simulink model "full_simulation"  (R2025b)
settings: Solver=VariableStepAuto  StopTime=2000
values from neighbouring files (symbols this model uses):
  s = sensors.gyro.scaleFactor    [detumbling_Simulation_cuerpo_ABC.m]    (also in pucp_orbit_propagator.m = z / r_norm; test_PUCP_1.m = z / r_norm)
undefined symbols (not defined in the file or in its folder): Adaptive_controler, deg, dow, eu, I, IAU, InitialCondition, K, k_bdot, Ley_adaptacion, P, rad, reference_euler, w_r, w_s
libraries: aerolibconvert2 x6, matrix_library x4, sharedtransform x3, aerolibutil x2, simulink_extras x2, aerolibtransform2 x1
settings Model: Creator=b_ant  LastModifiedBy=b_ant
settings ConfigComp: PLC_TargetIDE=codesys35  PLC_MultiTBSigbuilderTimeRange=off  PLC_FoldFBCallOutputVar=off  PLC_RemoveUnusedSSMethodCallArguments=off  PLC_UseCallOutputArgSyntax=off  PLC_EnableUnsignedAndDoubleTypes=off  PLC_EnableUDTSplitting=off  PLC_MaxFieldsInUDT=500.0  PLC_InlineEnumCastFunction=off  PLC_RTWMaxIdLength=31.0  PLC_RollThreshold=5.0  PLC_ActiveTab=0.0  PLC_EnableStringLiteralTB=on  PLC_Enable64bitIntSupport=off
settings SimscapeCC: SimscapeNominalValues="[{\"value\":\"1\",\"unit\":\"A\"},{\"value\":\"1\",\"unit\":\"bar\"},{\"value\":\"1\",\"unit\":\"cm^2\"},{\"value\":\"1\",\"unit\":\"cm^3/s\"},{\"value\":\"1\",\"unit\":\"kJ/kg\"},{\"value\":\"1\",\"unit\":\"kW\"},{\"value\":\"1\",\"unit\":\"l\"},{\"value\":\"1\",\"unit\":\"N\"},{\"value\":\"1\",\"unit\":\"N*m\"},{\"value\":\"1\",\"unit\":\"V\"},{\"value\":\"0.001\",\"unit\":\"Wb\"}]"  SimscapeLogType=all  SimscapeLogDataHistory=10000.0

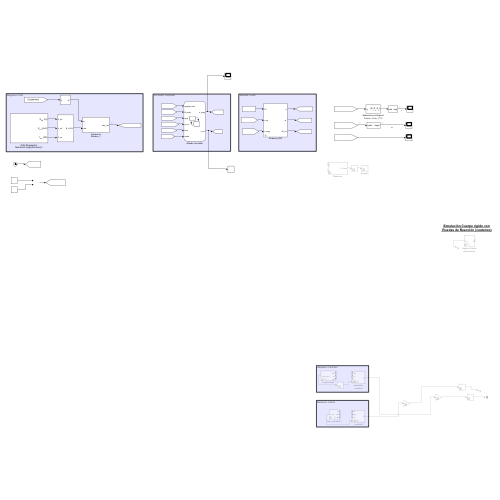
[thumbnail: Simulink's stored preview of the top-level diagram]
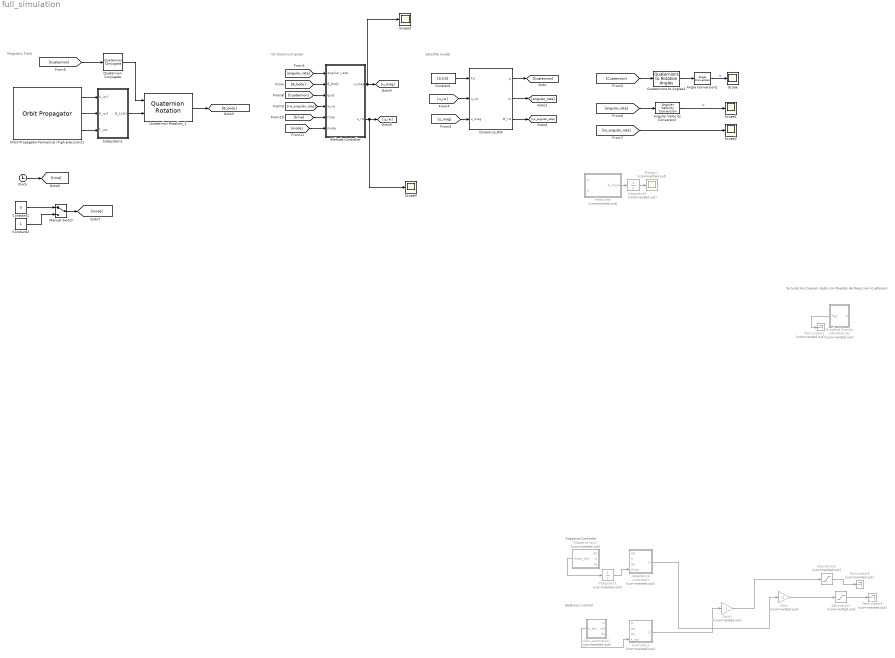
== system full_simulation ==
  note: Satellite model
  note: On board computer
  note: Magnetic Field
  note: Boskovic control
  note: Adaptive Controler
  note: Simulación Cuerpo rígido con
      | Ruedas de Reacción (cuatenos)
  Adaptative controler1 : Subsystem  Commented=on  mask{J=[1,1,1,0,0,0], lambda=1, kd=1}
      mask prompts: J "[Jcxx,Jcyy,Jczz,Jcxy,Jcxz,Jcyz]:"
      mask TypeOptions J: J/Value
      mask TypeOptions lambda: lambda/Value
      mask TypeOptions kd: Kd/Value
      mask DialogControl DescGroupVar Prompt: Adaptive controler
      mask DialogControl Control2 Prompt: Modeled inertia tensor:
      mask DialogControl H Prompt: Gains
  Adaptive law1 : Subsystem  Commented=on  mask{gamma=0.001, Lambda=1}
      mask TypeOptions gamma: gamma/Value
      mask TypeOptions Lambda: lambda/Value
  Angle Conversion2 : aerolibconvert2/Angle Conversion  IU=rad  OU=deg
  Angular Velocity Conversion : aerolibconvert2/Angular Velocity Conversion  IU=rad/s  OU=deg/s
  Attitude Controller : Stateflow chart  TreatAsAtomicUnit=on
  Clock : Clock
  Constant : Constant  Value=[0,0,0]
  Constant1 : Constant  Value=0
  Constant2 : Constant
  Controler1 : Subsystem  Commented=on  mask{delta=1, Umax=1.343*10^(-2)}
      mask TypeOptions delta: delta/Value
      mask TypeOptions Umax: Umax/Value
      mask DialogControl DescGroupVar Prompt: Boskovic Control
      mask DialogControl Control2 Prompt: Delta:
      mask DialogControl Control3 Prompt: Umax:
  Dinamica_RW : Subsystem  mask{I=I, Ang=eu, W=w_s, Wrw=w_r, dimensiones=dow}
      mask prompts: I "[Ix,Iy,Iz,Ixy,Ixz,Iyz] :"; Ang "[roll,pitch,yaw]:"; W "[Wx,Wy,Wz]"; Wrw "[Wrwx,Wrwy,Wrwz]"; dimensiones "[Ancho,Masa,Radio]:"
      mask TypeOptions I: I/Value
      mask TypeOptions Ang: Ang/Value
      mask TypeOptions W: W/Value
      mask TypeOptions Wrw: Wrw/Value
      mask TypeOptions dimensiones: dimentions/Value
      mask DialogControl Container3 Prompt: Tensor de Inercia
      mask DialogControl Container2 Prompt: Condiciones iniciales
      mask DialogControl Container4 Prompt: Ruedas de Reacción:
      mask DialogControl Control1 Prompt: Dimensiones:
  Energy1 : Scope  Commented=on
      settings: TimeSpan=10  ActiveDisplayYMinimum=0  ActiveDisplayYMaximum=2.75  DataLoggingVariableName=Energia3  DataLoggingSaveFormat=Array
  Gain : Gain  Commented=on  Gain=-1
  Gain1 : Gain  Commented=on  Gain=-1
  Gain_estimator1 : Subsystem  Commented=on  mask{delta=1, gamma=0.001, Umax=1.343*10^(-2), InitialCondition=1}
      mask prompts: InitialCondition "Simulink:blkprm_prompts:IntegratorInitCond"
      mask TypeOptions delta: delta/Value
      mask TypeOptions gamma: gamma/Value
      mask TypeOptions Umax: Umax/Value
      mask TypeOptions InitialCondition: Integrator/InitialCondition
      mask DialogControl DescGroupVar Prompt: Gain_estimator
      mask DialogControl Control2 Prompt: Gains:
      mask DialogControl Control3 Prompt: Initial Gain:
      mask DialogControl InitialCondition Prompt: Initial condition:
  Gradient Gravity disturbances : Subsystem  Commented=on  mask{J_tilde=[8.46,8.46,8.46,1.1,1.5,1.6]*10^(-3), rc=(6371+100)*10^(3), Drw=[0.015,0.025,0.043]}
      mask prompts: J_tilde "Satellite Inertia Tensor:"; rc "Distance from the center of the earth:"; Drw "Reaction wheels dimentions"
      mask TypeOptions J_tilde: J_tilde/Value
      mask TypeOptions rc: rc/Value
      mask TypeOptions Drw: dimentions/Value
      mask DialogControl DescGroupVar Prompt: Gravity gradient Torque
  Integrator1 : Integrator  Commented=on  InitialCondition=[1,1,1,0,0,0]
  Integrator3 : Integrator  Commented=on
  Manual Switch : ManualSwitch
  Measures : Subsystem  Commented=on
  Orbit Propagator Numerical (high precision)1 : OrbitPropagator  accelFrame=Fixed-frame  outportFrame=Fixed-frame  semiMajorAxis=orbit.semiMajorAxis  eccentricity=orbit.eccentricity  inclination=orbit.inclination  raan=orbit.rightAscensionOfAscendingNode  argPeriapsis=orbit.argumentOfPeriapsis  trueAnomaly=orbit.trueAnomaly  inertialPosition=[3649700.0 3308200.0 -4676600.0]  inertialVelocity=[-2750.8 6666.4 2573.4]  fixedPosition=[-4142689.0 -2676864.7 -4669861.6]  fixedVelocity=[1452.7 -6720.7 2568.1]  gravityModel=None  customR=3396200  customMu=4.305e13  customJ2=1.0826269e-03  customOmega=4.06125949e-3  outputTransform=on
  Quaternion Conjugate : aerolibutil/Quaternion Conjugate
  Quaternion Rotation_1 : aerolibutil/Quaternion Rotation
  Quaternions to Angles2 : sharedtransform/Quaternions to Rotation Angles  rotationOrder=ZYX  aMode=aMode
  Saturation1 : Saturate  Commented=on  UpperLimit=1.343*10^(-2)  LowerLimit=-1.343*10^(-2)
  Saturation2 : Saturate  Commented=on  UpperLimit=1.343*10^(-2)  LowerLimit=-1.343*10^(-2)
  Scope{,1..4} (5 alike) : Scope
      Scope settings: ActiveDisplayYMinimum=-23.210840938697004  ActiveDisplayYMaximum=43.99322143114955
      Scope1 settings: ActiveDisplayYMinimum=-0.62287287742311848  ActiveDisplayYMaximum=1.7831039675067617
      Scope2 settings: DataLoggingVariableName=ScopeData2
      Scope3 settings: ActiveDisplayYMinimum=-3.3528933558992531E-7  ActiveDisplayYMaximum=3.2851122357621673E-7  DataLoggingVariableName=ScopeData3
      Scope4 settings: ActiveDisplayYMinimum=-2.4173536825278268E-5  ActiveDisplayYMaximum=5.4003519984842569E-6  DataLoggingVariableName=ScopeData4
  Subsystem1 : Subsystem
  Terminator1 : Terminator  Commented=on
  Terminator4 : Terminator  Commented=on
  Terminator6 : Terminator  Commented=on
  wires:
  Quaternions to Angles2/1 -> Angle Conversion2/1
  Integrator3/1 -> Energy1/1
  Saturation2/1 -> Terminator6/1
  Integrator1/1 -> Adaptative controler1/4(theta)
  Controler1/1(U) -> Gain1/1
  Adaptive law1/1(theta_dot) -> Integrator1/1
  Gain/1 -> Saturation1/1
  Measures/1("K, theta") -> Integrator3/1
  Gain_estimator1/1(k_est) -> Controler1/4(K_est)
  Adaptative controler1/1(U) -> Gain/1
  Gain1/1 -> Saturation2/1
  Saturation1/1 -> Terminator4/1
  Angle Conversion2/1 -> Scope/1  "q"
  Gradient Gravity disturbances/1(Tgg) -> Terminator1/1
  Orbit Propagator Numerical (high precision)1/1 -> Subsystem1/1(X_icrf)
  Orbit Propagator Numerical (high precision)1/2 -> Subsystem1/2(V_icrf)
  Orbit Propagator Numerical (high precision)1/3 -> Subsystem1/3(T_utc)
  Subsystem1/1(B_LVLH) -> Quaternion Rotation_1/2
  [Cuaternion] -> Quaternion Conjugate/1
  Dinamica_RW/1(q) -> [Cuaternion]
  Dinamica_RW/2("w ") -> [angular_rate]
  Dinamica_RW/3(W_rw) -> [rw_angular_rate]
  Quaternion Rotation_1/1 -> [B_body]
  [B_body] -> Attitude Controller/2(B_body)
  [angular_rate] -> Attitude Controller/1(angular_rate)
  [Cuaternion] -> Quaternions to Angles2/1
  Attitude Controller/1(u_mag) -> Scope3/1, [u_mag]
  Attitude Controller/2(u_rw) -> [u_rw], Scope4/1
  Constant/1 -> Dinamica_RW/1(Td)
  [rw_angular_rate] -> Scope2/1
  Angular Velocity Conversion/1 -> Scope1/1  "w"
  Quaternion Conjugate/1 -> Quaternion Rotation_1/1
  [u_rw] -> Dinamica_RW/2(u_rw)
  [u_mag] -> Dinamica_RW/3(u_mag)
  [Cuaternion] -> Attitude Controller/3(quat)
  [rw_angular_rate] -> Attitude Controller/4(w_rw)
  Clock/1 -> [time]
  Constant1/1 -> Manual Switch/1
  Constant2/1 -> Manual Switch/2
  [time] -> Attitude Controller/5(time)
  Manual Switch/1 -> [mode]
  [mode] -> Attitude Controller/6(mode)
  [angular_rate] -> Angular Velocity Conversion/1

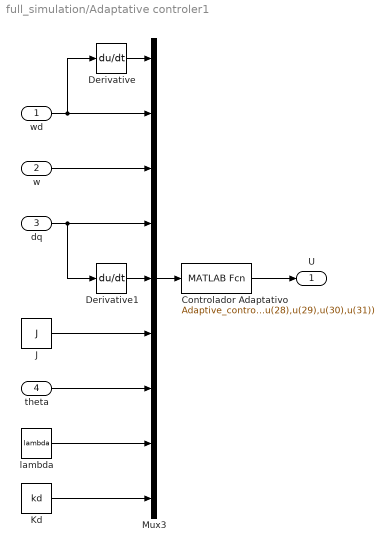
== system full_simulation/Adaptative controler1 ==
  wd : Inport
  w : Inport  Port=2
  dq : Inport  Port=3
  theta : Inport  Port=4
  Controlador Adaptativo : MATLABFcn  MATLABFcn=Adaptive_controler(u(1),u(2),u(3),u(4),u(5),u(6),u(7),u(8),u(9),u(10),u(11),u(12),u(13),u(14),u(15),u(16),u(17),u(18),u(19),u(20),u(21),u(22),u(23),u(24),u(25),u(26),u(27),u(28),u(29),u(30),u(31))
  Derivative : Derivative
  Derivative1 : Derivative
  J : Constant  Value=J
  Kd : Constant  Value=kd
  Mux3 : Mux  Inputs=9
  lambda : Constant  Value=lambda
  U : Outport
  wires:
  Mux3/1 -> Controlador Adaptativo/1
  Controlador Adaptativo/1 -> U/1
  Derivative/1 -> Mux3/1
  Kd/1 -> Mux3/9
  wd/1 -> Derivative/1, Mux3/2
  w/1 -> Mux3/3
  dq/1 -> Derivative1/1, Mux3/4
  Derivative1/1 -> Mux3/5
  J/1 -> Mux3/6
  theta/1 -> Mux3/7
  lambda/1 -> Mux3/8

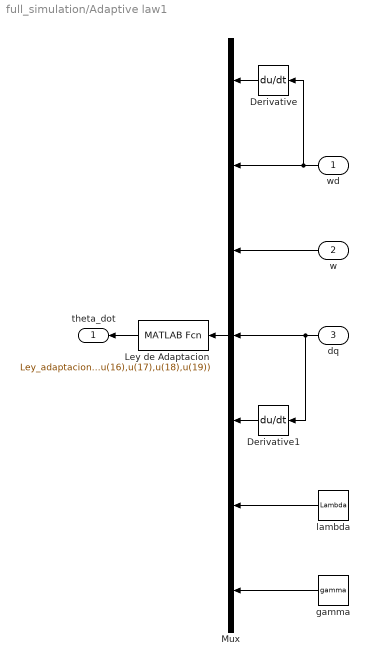
== system full_simulation/Adaptive law1 ==
  wd : Inport
  w : Inport  Port=2
  dq : Inport  Port=3
  Derivative : Derivative
  Derivative1 : Derivative
  Ley de Adaptacion : MATLABFcn  MATLABFcn=Ley_adaptacion(u(1),u(2),u(3),u(4),u(5),u(6),u(7),u(8),u(9),u(10),u(11),u(12),u(13),u(14),u(15),u(16),u(17),u(18),u(19))
  Mux : Mux  Inputs=7
  gamma : Constant  Value=gamma
  lambda : Constant  Value=Lambda
  theta_dot : Outport
  wires:
  wd/1 -> Derivative/1, Mux/2
  Mux/1 -> Ley de Adaptacion/1
  Ley de Adaptacion/1 -> theta_dot/1
  w/1 -> Mux/3
  dq/1 -> Derivative1/1, Mux/4
  Derivative1/1 -> Mux/5
  lambda/1 -> Mux/6
  gamma/1 -> Mux/7
  Derivative/1 -> Mux/1

== system full_simulation/Attitude Controller/Detumbling ==
  angular_rate : Inport
  B_body : Inport  Port=2
  quat : Inport  Port=3
  w_rw : Inport  Port=4
  Action Port : ActionPort
      settings: CopyFcn=Stateflow.SLINSF.SimulinkMan.removeBlockPreDeleteFcn  PreDeleteFcn=Stateflow.SLINSF.SimulinkMan.unsafePredeleteFcn
  B_dot_algorithm : Subsystem
  Terminator : Terminator
  Terminator1 : Terminator
  u_mag : Outport  VectorParamsAs1DForOutWhenUnconnected=off
  u_rw : Outport  Port=2  VectorParamsAs1DForOutWhenUnconnected=off
  wires:
  angular_rate/1 -> B_dot_algorithm/1(a)
  B_body/1 -> B_dot_algorithm/2(b)
  B_dot_algorithm/1(y) -> u_mag/1
  B_dot_algorithm/2(x) -> u_rw/1
  quat/1 -> Terminator/1
  w_rw/1 -> Terminator1/1

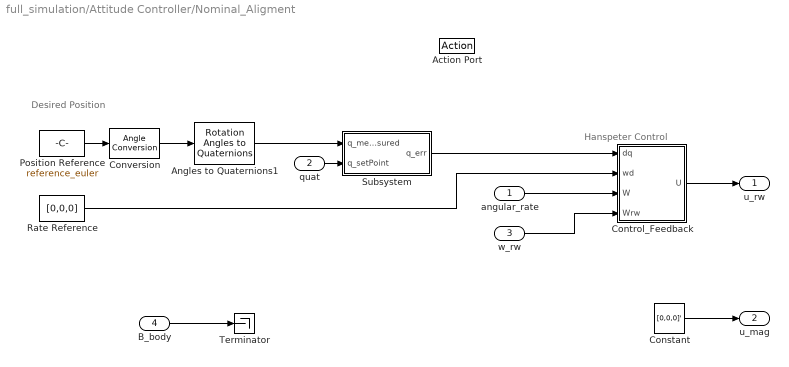
== system full_simulation/Attitude Controller/Nominal_Aligment ==
  note: Desired Position
  note: Hanspeter Control
  angular_rate : Inport
  quat : Inport  Port=2
  w_rw : Inport  Port=3
  B_body : Inport  Port=4
  Action Port : ActionPort
      settings: CopyFcn=Stateflow.SLINSF.SimulinkMan.removeBlockPreDeleteFcn  PreDeleteFcn=Stateflow.SLINSF.SimulinkMan.unsafePredeleteFcn
  Angles to Quaternions1 : sharedtransform/Rotation Angles to Quaternions  rotationOrder=ZYX  aMode=aMode
  Constant : Constant  Value=[0,0,0]'
  Control_Feedback : Subsystem  mask{Inertia=[1,1,1,0,0,0], P=P, K=K, dimentios=[0.00,0.0,0.0]}
      mask prompts: Inertia "[Ix,Iy,Iz,Ixy,Ixz,Iyz]:"; dimentios "[Grosor,Masa,Radio]:"
      mask TypeOptions Inertia: I/Value
      mask TypeOptions P: P/Value
      mask TypeOptions K: K/Value
      mask TypeOptions dimentios: dimentions/Value
      mask DialogControl ParameterGroupVar Prompt: Feedback Control
      mask DialogControl Control3 Prompt: Gains
      mask DialogControl Container2 Prompt: Reaction wheels
      mask DialogControl Control2 Prompt: Dimentions:
  Conversion : aerolibconvert2/Angle Conversion  IU=deg  OU=rad
  Position Reference : Constant  Value=reference_euler
  Rate Reference : Constant  Value=[0,0,0]
  Subsystem : Subsystem
  Terminator : Terminator
  u_rw : Outport  VectorParamsAs1DForOutWhenUnconnected=off
  u_mag : Outport  Port=2  VectorParamsAs1DForOutWhenUnconnected=off
  wires:
  Position Reference/1 -> Conversion/1
  Conversion/1 -> Angles to Quaternions1/1
  Angles to Quaternions1/1 -> Subsystem/1(q_measured)
  Subsystem/1(q_err) -> Control_Feedback/1(dq)
  quat/1 -> Subsystem/2(q_setPoint)
  angular_rate/1 -> Control_Feedback/3(W)
  w_rw/1 -> Control_Feedback/4(Wrw)
  Rate Reference/1 -> Control_Feedback/2(wd)
  Control_Feedback/1(U) -> u_rw/1
  Constant/1 -> u_mag/1
  B_body/1 -> Terminator/1

== system full_simulation/Attitude Controller/Settling ==
  angular_rate : Inport
  B_body : Inport  Port=2
  quat : Inport  Port=3
  w_rw : Inport  Port=4
  Action Port : ActionPort
      settings: CopyFcn=Stateflow.SLINSF.SimulinkMan.removeBlockPreDeleteFcn  PreDeleteFcn=Stateflow.SLINSF.SimulinkMan.unsafePredeleteFcn
  B_dot_algorithm : Subsystem
  Terminator : Terminator
  Terminator1 : Terminator
  u_mag : Outport  VectorParamsAs1DForOutWhenUnconnected=off
  u_rw : Outport  Port=2  VectorParamsAs1DForOutWhenUnconnected=off
  wires:
  quat/1 -> Terminator/1
  B_dot_algorithm/1(y) -> u_mag/1
  angular_rate/1 -> B_dot_algorithm/1(a)
  w_rw/1 -> Terminator1/1
  B_body/1 -> B_dot_algorithm/2(b)
  B_dot_algorithm/2(x) -> u_rw/1

== system full_simulation/Controler1 ==
  w : Inport
  wd : Inport  Port=2
  dq : Inport  Port=3
  K_est : Inport  Port=4
  Boskovic_control : MATLABFcn  MATLABFcn=Boskovic_control
  Mux : Mux  Inputs=6
  Umax : Constant  Value=Umax
  delta : Constant  Value=delta
  U : Outport
  wires:
  Boskovic_control/1 -> U/1
  Mux/1 -> Boskovic_control/1
  Umax/1 -> Mux/6
  K_est/1 -> Mux/5
  delta/1 -> Mux/4
  dq/1 -> Mux/3
  wd/1 -> Mux/2
  w/1 -> Mux/1

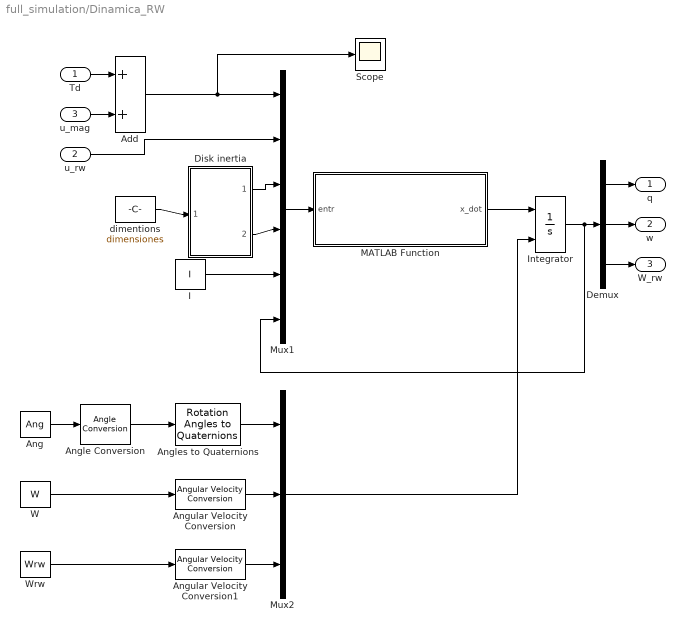
== system full_simulation/Dinamica_RW ==
  Td : Inport  PortDimensions=[3,1]
  u_rw : Inport  Port=2  PortDimensions=[3,1]
  u_mag : Inport  Port=3  PortDimensions=[3,1]
  Add : Sum
  Ang : Constant  Value=Ang
  Angle Conversion : aerolibconvert2/Angle Conversion  IU=deg  OU=rad
  Angles to Quaternions : sharedtransform/Rotation Angles to Quaternions  rotationOrder=ZYX  aMode=aMode
  Angular Velocity Conversion : aerolibconvert2/Angular Velocity Conversion  IU=deg/s  OU=rad/s
  Angular Velocity Conversion1 : aerolibconvert2/Angular Velocity Conversion  IU=deg/s  OU=rad/s
  Demux : Demux  Outputs=3
  Disk inertia : Subsystem
  I : Constant  Value=I
  Integrator : Integrator  InitialConditionSource=external  InitialCondition=InitialCondition
  MATLAB Function : MATLAB Function  TreatAsAtomicUnit=on
  Mux1 : Mux  Inputs=6
  Mux2 : Mux  Inputs=3
  Scope : Scope
      settings: ActiveDisplayYMinimum=-1  ActiveDisplayYMaximum=1  DataLoggingVariableName=ScopeData5
  W : Constant  Value=W
  Wrw : Constant  Value=Wrw
  dimentions : Constant  Value=dimensiones
  q : Outport  PortDimensions=[4,1]
  "w " : Outport  Port=2  PortDimensions=[3,1]
  W_rw : Outport  Port=3  PortDimensions=[3,1]
  wires:
  Demux/1 -> q/1
  Demux/3 -> W_rw/1
  Demux/2 -> "w "/1
  MATLAB Function/1(x_dot) -> Integrator/1
  Mux1/1 -> MATLAB Function/1(entr)
  u_rw/1 -> Mux1/2
  I/1 -> Mux1/5
  Mux2/1 -> Integrator/2
  Angular Velocity Conversion1/1 -> Mux2/3
  Angular Velocity Conversion/1 -> Mux2/2
  Angle Conversion/1 -> Angles to Quaternions/1
  Ang/1 -> Angle Conversion/1
  Wrw/1 -> Angular Velocity Conversion1/1
  Angles to Quaternions/1 -> Mux2/1
  Integrator/1 -> Mux1/6, Demux/1
  W/1 -> Angular Velocity Conversion/1
  dimentions/1 -> Disk inertia/1(Dimentions)
  Disk inertia/1(Irw_per) -> Mux1/3
  Disk inertia/2(Irw_par) -> Mux1/4
  Add/1 -> Scope/1, Mux1/1
  Td/1 -> Add/1
  u_mag/1 -> Add/2

== system full_simulation/Gain_estimator1 ==
  w : Inport
  wd : Inport  Port=2
  dq : Inport  Port=3
  Gain_estimator : MATLABFcn  MATLABFcn=Gain_estimator
  Integrator : Integrator  InitialCondition=InitialCondition
  Mux : Mux  Inputs=7
  Umax : Constant  Value=Umax
  delta : Constant  Value=delta
  gamma : Constant  Value=gamma
  k_est : Outport
  wires:
  Gain_estimator/1 -> Integrator/1
  Mux/1 -> Gain_estimator/1
  Integrator/1 -> Mux/6, k_est/1
  Umax/1 -> Mux/7
  gamma/1 -> Mux/5
  delta/1 -> Mux/4
  dq/1 -> Mux/3
  wd/1 -> Mux/2
  w/1 -> Mux/1

== system full_simulation/Gradient Gravity disturbances ==
  q : Inport
  Disk inertia : Subsystem
  Gravity disturbances : MATLABFcn  MATLABFcn=T_disturbances
  J_tilde : Constant  Value=J_tilde
  Mux3 : Mux
  Terminator2 : Terminator
  dimentions : Constant  Value=Drw
  rc : Constant  Value=rc
  Tgg : Outport
  wires:
  dimentions/1 -> Disk inertia/1(Dimentions)
  rc/1 -> Mux3/3
  J_tilde/1 -> Mux3/1
  Mux3/1 -> Gravity disturbances/1
  Disk inertia/1(Irw_per) -> Mux3/4
  Disk inertia/2(Irw_par) -> Terminator2/1
  q/1 -> Mux3/2
  Gravity disturbances/1 -> Tgg/1

== system full_simulation/Measures ==
  q : Inport
  u : Inport  Port=2
  Measure : MATLABFcn  MATLABFcn=Measures
  Mux3 : Mux  Inputs=2
  "K, theta" : Outport
  wires:
  Measure/1 -> "K, theta"/1
  Mux3/1 -> Measure/1
  q/1 -> Mux3/1
  u/1 -> Mux3/2

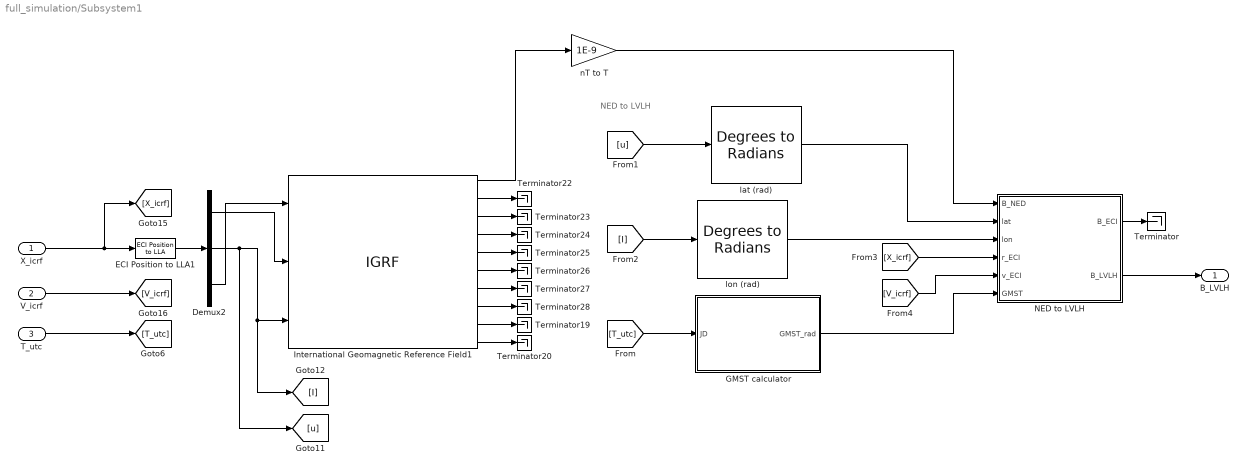
== system full_simulation/Subsystem1 ==
  note: NED to LVLH
  X_icrf : Inport
  V_icrf : Inport  Port=2
  T_utc : Inport  Port=3
  " NED to LVLH" : MATLAB Function  TreatAsAtomicUnit=on
  Demux2 : Demux  Outputs=3
  ECI Position to LLA1 : aerolibtransform2/ECI Position to LLA  red=IAU-2000/2006  year=2020  month=January  day=1  hour=0  min=0  sec=0  deltaT=None  errorflag=Error  extraparamflag=off  eunits=Metric (MKS)  earthmodel=WGS84  flat=1/298.257223563  eqradius=6378137
      settings: AttributesFormatString=%<red>
  GMST calculator : MATLAB Function  TreatAsAtomicUnit=on
  International Geomagnetic Reference Field1 : IGRF  time_in=off  month=January  day=1  year=2020
      settings: AttributesFormatString=%<generation>
  Terminator{,19..20,22..28} (10 alike) : Terminator
  lat (rad) : simulink_extras/Transformations/Degrees to Radians
  lon (rad) : simulink_extras/Transformations/Degrees to Radians
  nT to T : Gain  Gain=1E-9
  B_LVLH : Outport
  wires:
  International Geomagnetic Reference Field1/3 -> Terminator23/1
  Demux2/2 -> [I], International Geomagnetic Reference Field1/3, [u]
  International Geomagnetic Reference Field1/7 -> Terminator27/1
  " NED to LVLH"/1(B_ECI) -> Terminator/1
  [I] -> lon (rad)/1
  V_icrf/1 -> [V_icrf]
  lat (rad)/1 -> " NED to LVLH"/2(lat)
  International Geomagnetic Reference Field1/9 -> Terminator19/1
  International Geomagnetic Reference Field1/10 -> Terminator20/1
  ECI Position to LLA1/1 -> Demux2/1
  [X_icrf] -> " NED to LVLH"/4(r_ECI)
  [u] -> lat (rad)/1
  X_icrf/1 -> ECI Position to LLA1/1, [X_icrf]
  International Geomagnetic Reference Field1/5 -> Terminator25/1
  International Geomagnetic Reference Field1/8 -> Terminator28/1
  T_utc/1 -> [T_utc]
  " NED to LVLH"/2(B_LVLH) -> B_LVLH/1
  nT to T/1 -> " NED to LVLH"/1(B_NED)
  International Geomagnetic Reference Field1/2 -> Terminator22/1
  [T_utc] -> GMST calculator/1(JD)
  GMST calculator/1(GMST_rad) -> " NED to LVLH"/6(GMST)
  International Geomagnetic Reference Field1/6 -> Terminator26/1
  International Geomagnetic Reference Field1/4 -> Terminator24/1
  lon (rad)/1 -> " NED to LVLH"/3(lon)
  [V_icrf] -> " NED to LVLH"/5(v_ECI)
  Demux2/3 -> International Geomagnetic Reference Field1/1
  International Geomagnetic Reference Field1/1 -> nT to T/1
  Demux2/1 -> International Geomagnetic Reference Field1/2

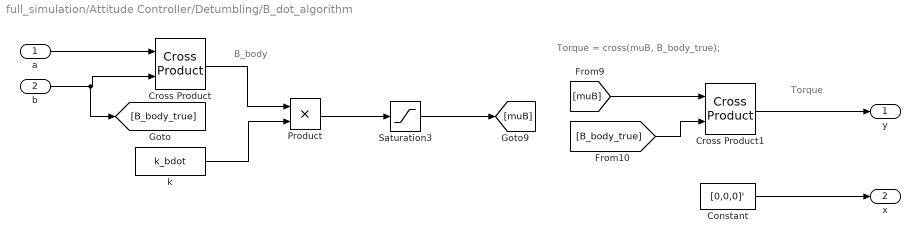
== system full_simulation/Attitude Controller/Detumbling/B_dot_algorithm ==
  note: Torque = cross(muB, B_body_true);
  note: B_body
  note: Torque
  a : Inport
  b : Inport  Port=2
  Constant : Constant  Value=[0,0,0]'
  Cross Product : matrix_library/Cross Product
  Cross Product1 : matrix_library/Cross Product
  Product : Product
  Saturation3 : Saturate  UpperLimit=Inf  LowerLimit=-Inf
  k : Constant  Value=k_bdot
  y : Outport
  x : Outport  Port=2
  wires:
  Cross Product1/1 -> y/1
  Saturation3/1 -> [muB]
  [muB] -> Cross Product1/1
  [B_body_true] -> Cross Product1/2
  b/1 -> [B_body_true], Cross Product/2
  k/1 -> Product/2
  Cross Product/1 -> Product/1
  Product/1 -> Saturation3/1
  a/1 -> Cross Product/1
  Constant/1 -> x/1

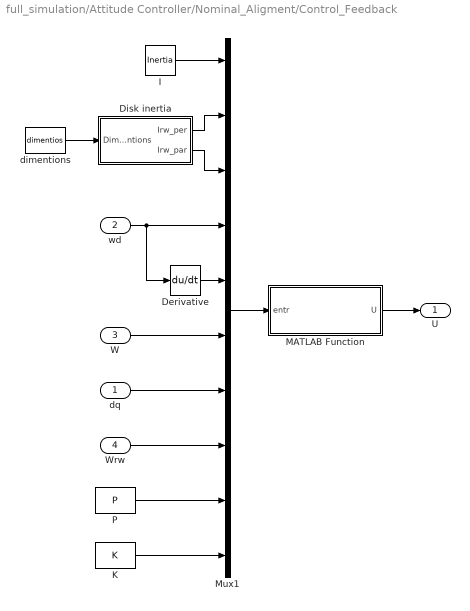
== system full_simulation/Attitude Controller/Nominal_Aligment/Control_Feedback ==
  dq : Inport  PortDimensions=[4,1]
  wd : Inport  Port=2  PortDimensions=[3,1]
  W : Inport  Port=3  PortDimensions=[3,1]
  Wrw : Inport  Port=4  PortDimensions=[3,1]
  Derivative : Derivative
  Disk inertia : Subsystem
  I : Constant  Value=Inertia
  K : Constant  Value=K
  MATLAB Function : MATLAB Function  TreatAsAtomicUnit=on
  Mux1 : Mux  Inputs=10
  P : Constant  Value=P
  dimentions : Constant  Value=dimentios
  U : Outport  PortDimensions=[3,1]
  wires:
  Derivative/1 -> Mux1/5
  Mux1/1 -> MATLAB Function/1(entr)
  I/1 -> Mux1/1
  MATLAB Function/1(U) -> U/1
  W/1 -> Mux1/6
  Wrw/1 -> Mux1/8
  dq/1 -> Mux1/7
  wd/1 -> Derivative/1, Mux1/4
  dimentions/1 -> Disk inertia/1(Dimentions)
  Disk inertia/1(Irw_per) -> Mux1/2
  Disk inertia/2(Irw_par) -> Mux1/3
  K/1 -> Mux1/10
  P/1 -> Mux1/9

== system full_simulation/Attitude Controller/Nominal_Aligment/Subsystem ==
  q_measured : Inport
  q_setPoint : Inport  Port=2
  Demux : Demux
  Demux1 : Demux
  MATLAB Function : MATLAB Function  TreatAsAtomicUnit=on
  q_err : Outport
  wires:
  Demux1/2 -> MATLAB Function/6(q1)
  Demux1/3 -> MATLAB Function/7(q2)
  Demux1/4 -> MATLAB Function/8(q3)
  Demux/3 -> MATLAB Function/3(qm2)
  Demux/4 -> MATLAB Function/4(qm3)
  Demux/1 -> MATLAB Function/1(qm0)
  Demux/2 -> MATLAB Function/2(qm1)
  Demux1/1 -> MATLAB Function/5(q0)
  q_measured/1 -> Demux/1
  q_setPoint/1 -> Demux1/1
  MATLAB Function/1(q_err) -> q_err/1

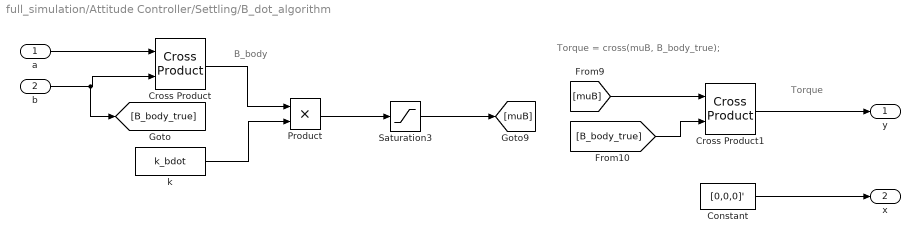
== system full_simulation/Attitude Controller/Settling/B_dot_algorithm ==
  note: Torque = cross(muB, B_body_true);
  note: B_body
  note: Torque
  a : Inport
  b : Inport  Port=2
  Constant : Constant  Value=[0,0,0]'
  Cross Product : matrix_library/Cross Product
  Cross Product1 : matrix_library/Cross Product
  Product : Product
  Saturation3 : Saturate  UpperLimit=Inf  LowerLimit=-Inf
  k : Constant  Value=k_bdot
  y : Outport
  x : Outport  Port=2
  wires:
  Cross Product1/1 -> y/1
  Saturation3/1 -> [muB]
  [muB] -> Cross Product1/1
  [B_body_true] -> Cross Product1/2
  b/1 -> [B_body_true], Cross Product/2
  k/1 -> Product/2
  Cross Product/1 -> Product/1
  Product/1 -> Saturation3/1
  a/1 -> Cross Product/1
  Constant/1 -> x/1

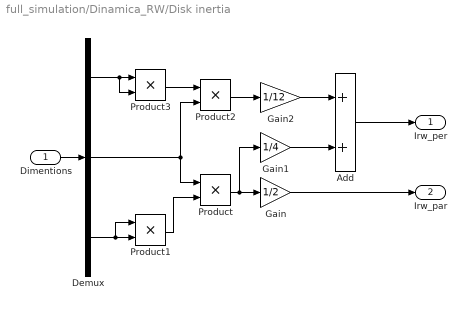
== system full_simulation/Dinamica_RW/Disk inertia ==
  Dimentions : Inport
  Add : Sum
  Demux : Demux  Outputs=3
  Gain : Gain  Gain=1/2
  Gain1 : Gain  Gain=1/4
  Gain2 : Gain  Gain=1/12
  Product{,1..3} (4 alike) : Product
  Irw_per : Outport
  Irw_par : Outport  Port=2
  wires:
  Product3/1 -> Product2/1
  Gain2/1 -> Add/1
  Product/1 -> Gain1/1, Gain/1
  Add/1 -> Irw_per/1
  Gain1/1 -> Add/2
  Product1/1 -> Product/2
  Gain/1 -> Irw_par/1
  Demux/1 -> Product3/2, Product3/1
  Product2/1 -> Gain2/1
  Demux/2 -> Product/1, Product2/2
  Dimentions/1 -> Demux/1
  Demux/3 -> Product1/1, Product1/2

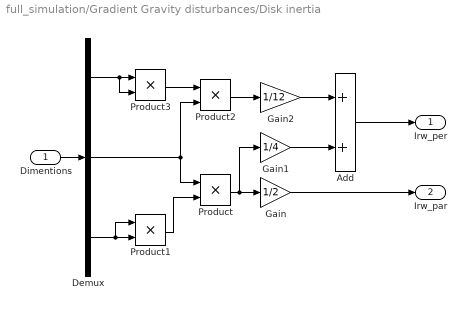
== system full_simulation/Gradient Gravity disturbances/Disk inertia ==
  Dimentions : Inport
  Add : Sum
  Demux : Demux  Outputs=3
  Gain : Gain  Gain=1/2
  Gain1 : Gain  Gain=1/4
  Gain2 : Gain  Gain=1/12
  Product{,1..3} (4 alike) : Product
  Irw_per : Outport
  Irw_par : Outport  Port=2
  wires:
  Product3/1 -> Product2/1
  Gain2/1 -> Add/1
  Product/1 -> Gain1/1, Gain/1
  Add/1 -> Irw_per/1
  Gain1/1 -> Add/2
  Product1/1 -> Product/2
  Gain/1 -> Irw_par/1
  Demux/1 -> Product3/2, Product3/1
  Product2/1 -> Gain2/1
  Demux/2 -> Product/1, Product2/2
  Dimentions/1 -> Demux/1
  Demux/3 -> Product1/1, Product1/2

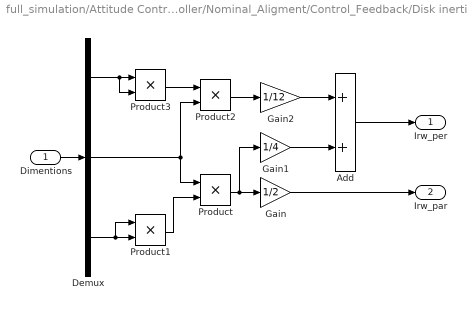
== system full_simulation/Attitude Controller/Nominal_Aligment/Control_Feedback/Disk inertia ==
  Dimentions : Inport
  Add : Sum
  Demux : Demux  Outputs=3
  Gain : Gain  Gain=1/2
  Gain1 : Gain  Gain=1/4
  Gain2 : Gain  Gain=1/12
  Product{,1..3} (4 alike) : Product
  Irw_per : Outport
  Irw_par : Outport  Port=2
  wires:
  Product3/1 -> Product2/1
  Gain2/1 -> Add/1
  Product/1 -> Gain1/1, Gain/1
  Add/1 -> Irw_per/1
  Gain1/1 -> Add/2
  Product1/1 -> Product/2
  Gain/1 -> Irw_par/1
  Demux/1 -> Product3/2, Product3/1
  Product2/1 -> Gain2/1
  Demux/2 -> Product/1, Product2/2
  Dimentions/1 -> Demux/1
  Demux/3 -> Product1/1, Product1/2

== matlab function full_simulation/Dinamica_RW/MATLAB Function ==
  data: entr input; x_dot output
function x_dot  = cubesat_rigid_dynamics_with_rw(entr)
% EQUATION_STATE_RW Calculates the state derivatives for a satellite with reaction wheels.
%
%   Syntax:
%       x_dot = EQUATION_STATE_RW(entr)
%
%   Description:
%       Computes the quaternion kinematics and rigid body dynamics based on 
%       Markley & Crassidis (2014). This model accounts for the interaction 
%       between the main spacecraft hub and three reaction wheels aligned with 
%       the body axes.
%
%   INPUTS (entr): 24-element input vector:
%       [1:3]   Td      : External disturbance torque [Nm]
%       [4:6]   U       : Control torque applied to the wheels [Nm]
%       [7]     Irw_per : Wheel inertia (perpendicular to the spin axis) [kg*m^2]
%       [8]     Irw_par : Wheel inertia (parallel to the spin axis/spin inertia) [kg*m^2]
%       [9:14]  Inertia : Components of the J_tilde tensor (Hub without wheels)
%       [15:18] q       : Current attitude quaternion [q0, q1, q2, q3]
%       [19:21] w       : Body angular velocity vector [rad/s]
%       [22:24] Wrw     : Relative angular velocity of the reaction wheels [rad/s]
%
%   OUTPUTS:
%       x_dot : State derivative vector [q_dot(4); w_dot(3); wrw_dot(3)]

% --- 1. Variable Extraction and Definition ---
Td = [entr(1),entr(2),entr(3)]';   
U  = [entr(4),entr(5),entr(6)]';    
Irw_per = entr(7);                 
Irw_par = entr(8);                 

% Construct the symmetric inertia tensor of the rigid body (J_tilde)
J_tilde = [entr(9),  entr(12), entr(13);
    entr(12), entr(10), entr(14);
    entr(13), entr(14), entr(11)];

% Wheel inertia matrix and General Inertia Tensor (Eq. 3.146)
R = diag(Irw_par * ones(1,3));             
J = J_tilde + diag(2 * Irw_per * ones(1,3));   

% --- 2. Current State Vectors ---
q   = [entr(15),entr(16),entr(17),entr(18)]'; % Attitude quaternion
w   = [entr(19),entr(20),entr(21)]'; % Body angular rate
Wrw = [entr(22),entr(23),entr(24)]'; % Reaction wheel angular rate

% --- 3. Quaternion Kinematics ---
% Based on the Xi propagation matrix (Eq. 2.88 from Markley & Crassidis)
% Maps angular velocity to the rate of change of orientation.
Xi = [-q(2), -q(3), -q(4);
    q(1), -q(4),  q(3);
    q(4),  q(1), -q(2);
    -q(3),  q(2),  q(1)]; 

% x1_dot: Quaternion derivative (q_dot) - Eq. 3.21
x1_dot = 0.5 * Xi * w;                                  

% --- 4. Attitude Dynamics (Euler's Equations) ---
% x2_dot: Body angular acceleration (w_dot) - Eq. 3.147
% Derived from the conservation of total angular momentum: H = Jw + R(w + Wrw)
% This accounts for the gyroscopic coupling and torque exchange.
%x2_dot = J \ (Td - U - cross(w, J*w + R*(w + Wrw)));      
x2_dot = J \ (Td - U - cross(w, J*w));      

% --- 5. Reaction Wheel Dynamics ---
% x3_dot: Relative angular acceleration of the wheels (Wrw_dot)
% Represents the internal acceleration of the wheel relative to the hub.
%x3_dot = (R \ U) - x2_dot;                   
x3_dot = [0,0,0]';                   

% --- 6. Assemble State Derivative Vector ---
x_dot = [x1_dot; x2_dot; x3_dot];
end

== matlab function full_simulation/Attitude Controller/Nominal_Aligment/Subsystem/MATLAB Function ==
  data: qm0 input; q_err output; qm1 input; qm2 input; qm3 input; q0 input; q1 input; q2 input; q3 input
function q_err  = quaternion_error(qm0, qm1, qm2, qm3, q0, q1, q2, q3)
% QUATERNION_ERROR: Calculates the rotation error between two quaternions.
%   [q_err] = QUATERNION_ERROR(qm0, qm1, qm2, qm3, q0, q1, q2, q3) computes 
%   the relative error quaternion representing the rotation required to 
%   transform the measured orientation (qm) into the desired orientation (q).
%
%   INPUTS:
%       qm0, qm1, qm2, qm3 : Components of the measured quaternion (scalar q0, vector q1-3).
%       q0, q1, q2, q3     : Components of the desired (reference) quaternion.
%
%   OUTPUTS:
%       q_err              : [4x1] Column vector containing the error quaternion [q0_e; q1_e; q2_e; q3_e].
%
%   MATHEMATICAL NOTES:
%   This function implements the quaternion product $q_{err} = q_m^* \otimes q$, 
%   where $q_m^*$ is the conjugate of the measured quaternion. It utilizes 
%   the $\Xi$-matrix (skew-symmetric auxiliary matrix) to perform the 
%   calculation via matrix multiplication:
%   q_err = [qm' * q; Xi' * q]

% 1. Define column vectors from input components
q  = [q0, q1, q2, q3]';
qm = [qm0, qm1, qm2, qm3]';

% 2. Construct the Xi matrix (Kinematic coupling matrix)
% This matrix maps the relationship between quaternion rates and angular velocity,
% or in this case, facilitates the Hamilton product in matrix form.
Xi = [-qm1, -qm2, -qm3;
    qm0, -qm3,  qm2;
    qm3,  qm0, -qm1;
    -qm2,  qm1,  qm0];

% 3. Calculate error quaternion components
% q13_err: The vector part (representing the rotation axis and sin(theta/2))
q13_err = Xi' * q;

% q0_err: The scalar part (representing cos(theta/2))
q0_err = qm' * q;

% 4. Assemble the output vector
q_err = [q0_err; q13_err];

end

== matlab function full_simulation/Attitude Controller/Nominal_Aligment/Control_Feedback/MATLAB Function ==
  data: entr input; U output
function U  = ControlFeedback_rw(entr)
% CONTROLFEEDBACK_RW Nonlinear Lyapunov-based Feedback Control for Reaction Wheels.
%
%   Syntax:
%       U = CONTROLFEEDBACK_RW(entr)
%
%   Description:
%       Computes the required control torque (U) to be applied to the reaction 
%       wheels. This law ensures asymptotic stability by canceling non-linear 
%       gyroscopic terms and implementing a PD-like tracking control.
%
%   INPUTS (entr): 26-element input vector:
%       [1:6]   Inertia : Unique components of the J_tilde tensor (Hub only).
%       [7]     Irw_per : Wheel inertia (perpendicular to spin axis).
%       [8]     Irw_par : Wheel inertia (parallel to spin axis).
%       [9:11]  Wr      : Reference (desired) angular velocity [rad/s].
%       [12:14] Wr_dot  : Reference angular acceleration [rad/s^2].
%       [15:17] W       : Current body angular velocity [rad/s].
%       [18]    dq0     : Scalar part of the error quaternion (not used in U).
%       [19:21] dq13    : Vector part of the error quaternion (Vectorial error).
%       [22:24] Wrw     : Relative angular velocity of reaction wheels [rad/s].
%       [25]    P       : Proportional gain (Damping for angular rate error).
%       [26]    K       : Stiffness gain (Proportional for attitude error).
%
%   OUTPUTS:
%       U       : [3x1] Control torque vector to be commanded to the motors [Nm].

% --- 1. Variable Definitions and Tensor Construction ---
% Reconstruct the symmetric inertia tensor J_tilde
J_tilde = [entr(1), entr(4), entr(5);
    entr(4), entr(2), entr(6);
    entr(5), entr(6), entr(3)];

Irw_per = entr(7);
Irw_par = entr(8);

% Reference and Current States
Wr     = [entr(9),entr(10),entr(11)]';
Wr_dot = [entr(12),entr(13),entr(14)]';                        
W      = [entr(15),entr(16),entr(17)]';
dq13   = [entr(19),entr(20),entr(21)]'; % Attitude error vector
Wrw    = [entr(22),entr(23),entr(24)]'; % Reaction wheel speeds

% Control Gains
P = entr(25);
K = entr(26);

% --- 2. Mathematical Calculations ---
% General Inertia Tensor (Including wheel housing contributions)
J = J_tilde + diag(2 * Irw_per * ones(1,3));   

% Angular Rate Error (We = W_actual - W_reference)
dW = W - Wr;                               

% Parallel Inertia Matrix of the wheels
R = diag(Irw_par * ones(1,3));             

% --- 3. Control Law (Feedback Linearization) ---
% The law consists of three main parts:
% 1. Proportional/Derivative tracking: P*dW + K*dq13
% 2. Gyroscopic compensation: -skew(W)*(J*W + R*(W + Wrw))
% 3. Reference acceleration tracking: -J*(Wr_dot - skew(W)*Wr)

U = P*dW + K*dq13 - skew(W)*(J*W + R*(W + Wrw)) - J*(Wr_dot - skew(W)*Wr);
end

== matlab function full_simulation/Subsystem1/ NED to LVLH ==
  data: B_NED input; B_ECI output; lat input; lon input; r_ECI input; v_ECI input; GMST input; B_LVLH output
function [B_ECI, B_LVLH] = fcn(B_NED, lat, lon, r_ECI, v_ECI, GMST)
% FCN Performs coordinate transformation of the Magnetic Field vector.
%
%   Syntax:
%       [B_ECI, B_LVLH] = fcn(B_NED, lat, lon, r_ECI, v_ECI, GMST)
%
%   Description:
%       Transforms the magnetic field vector from the local North-East-Down (NED) 
%       frame to the Earth-Centered Inertial (ECI) frame, and finally to the 
%       Local-Vertical Local-Horizontal (LVLH) frame (X: Velocity, Z: Nadir).
%
%   INPUTS:
%       B_NED  : Magnetic field vector in NED coordinates [3x1] (from IGRF).
%       lat    : Geodetic latitude [rad].
%       lon    : Geodetic longitude [rad].
%       r_ECI  : Satellite position vector in ECI frame [m].
%       v_ECI  : Satellite velocity vector in ECI frame [m/s].
%       GMST   : Greenwich Mean Sidereal Time [rad].
%
%   OUTPUTS:
%       B_ECI  : Magnetic field vector in ECI frame.
%       B_LVLH : Magnetic field vector in LVLH frame (Reference for attitude).

% --- 1. NED to ECEF Transformation ---
% Converts the local tangent plane vector (NED) to the Earth-Centered 
% Earth-Fixed (ECEF) rotating frame.
DCM_NED2ECEF = [-sin(lat)*cos(lon), -sin(lon), -cos(lat)*cos(lon);
    -sin(lat)*sin(lon),  cos(lon), -cos(lat)*sin(lon);
    cos(lat),           0,         -sin(lat)        ];
B_ECEF = DCM_NED2ECEF * B_NED;

% --- 2. ECEF to ECI Transformation ---
% Rotates the vector from the rotating Earth frame (ECEF) to the 
% inertial frame (ECI) using the Sidereal Time.
DCM_ECEF2ECI = [cos(GMST), -sin(GMST), 0;
    sin(GMST),  cos(GMST), 0;
    0,          0,         1];
B_ECI = DCM_ECEF2ECI * B_ECEF;

% --- 3. ECI to LVLH Transformation (X: Velocity-aligned, Z: Nadir) ---
% Construction of an orthonormal basis for the LVLH frame:

% Z-axis (Nadir): Pointing towards the center of the Earth.
z_hat = -r_ECI / norm(r_ECI); 

% Y-axis (Orbit Normal): Opposite to the angular momentum vector.
% Defined to ensure a right-handed system with Z pointing down.
h_vec = cross(r_ECI, v_ECI);
y_hat = -h_vec / norm(h_vec);

% X-axis (Along-track): Aligned with the velocity direction in the local horizontal.
% Guaranteed to be orthogonal to Y and Z.
x_hat = cross(y_hat, z_hat);

% Direction Cosine Matrix (DCM) from ECI to LVLH
DCM_ECI2LVLH = [x_hat'; y_hat'; z_hat'];

% --- 4. Final Output Projection ---
% Projects the inertial magnetic field into the satellite's local frame.
B_LVLH = DCM_ECI2LVLH * B_ECI;
end

== matlab function full_simulation/Subsystem1/GMST calculator ==
  data: JD input; GMST_rad output
function GMST_rad = fcn(JD)
% Entrada: JD = Fecha Juliana
% Salida: GMST en radianes

T = (JD - 2451545.0) / 36525.0;  
GMST_seg = 67310.54841 + ...
           (876600*3600 + 8640184.812866)*T + ...
           0.093104*T^2 - ...
           6.2e-6*T^3;

GMST_deg = mod(GMST_seg / 240.0, 360.0);

GMST_rad = deg2rad(GMST_deg);
end

== stateflow chart full_simulation/Attitude Controller ==
  state Nominal_Aligment
  state Detumbling
  state Settling
  (default) -> Detumbling
  Settling -> Nominal_Aligment : [after(120,sec)]
  Detumbling -> Settling : [(norm(angular_rate) < 1*pi/180) && after(5, sec)]
  data: sf_internal_action_state_placeholder_data local double size=1 =0; sf_internal_action_state_placeholder_data local double size=1 =0; sf_internal_action_state_placeholder_data local double size=1 =0; angular_rate input size=[3,1]; u_mag output size=[3,1]; B_body input size=[3,1]; u_rw output size=[3,1]; quat input size=[4,1]; w_rw input size=[3,1]; time input size=1; mode input size=1
